simulink model "drone_sine_text"  (R2019a)
settings: Solver=VariableStepAuto  StartTime=0.0  StopTime=inf  RelTol=1e-3
libraries: robotlib x2, aerolibanimutils x1
settings Model: Creator=flying  LastModifiedBy=flying

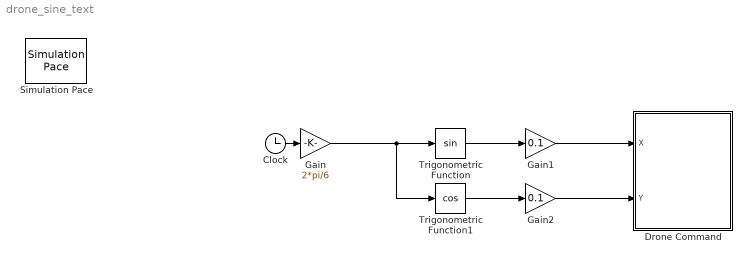
== system drone_sine_text ==
  Clock : Clock
  Drone Command : Subsystem
  Gain : Gain  Gain=2*pi/6
  Gain1 : Gain  Gain=0.1
  Gain2 : Gain  Gain=0.1
  Simulation Pace : aerolibanimutils/Simulation Pace  SimulationPace=1  SleepMode=Auto  OutputPaceError=off  SampleTime=1/30
  Trigonometric Function : Trigonometry
  Trigonometric Function1 : Trigonometry  Operator=cos
  wires:
  Gain/1 -> Trigonometric Function1/1, Trigonometric Function/1
  Clock/1 -> Gain/1
  Trigonometric Function/1 -> Gain1/1
  Trigonometric Function1/1 -> Gain2/1
  Gain1/1 -> Drone Command/1(X)
  Gain2/1 -> Drone Command/2(Y)

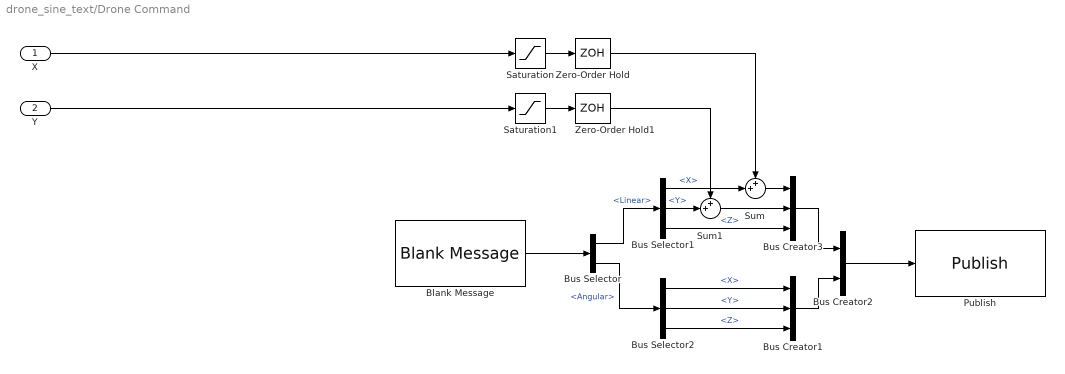
== system drone_sine_text/Drone Command ==
  X : Inport
  Y : Inport  Port=2
  Blank Message : robotlib/Blank Message  messageClass=Message  entityType=geometry_msgs/Twist  messageType=geometry_msgs/Twist  SampleTime=0.0333333333333333333333333
      settings: SourceProductBaseCode=RO
  Bus Creator1 : BusCreator  Inputs=3  OutDataTypeStr=Bus: SL_Bus_drone_sine_text_geometry_msgs_Vector3  NonVirtualBus=on
      settings: InheritFromInputs=off
  Bus Creator2 : BusCreator  Inputs=2  OutDataTypeStr=Bus: SL_Bus_drone_sine_text_geometry_msgs_Twist  NonVirtualBus=on
      settings: InheritFromInputs=off
  Bus Creator3 : BusCreator  Inputs=3  OutDataTypeStr=Bus: SL_Bus_drone_sine_text_geometry_msgs_Vector3  NonVirtualBus=on
      settings: InheritFromInputs=off
  Bus Selector : BusSelector  OutputSignals=Linear,Angular
  Bus Selector1 : BusSelector  OutputSignals=X,Y,Z
  Bus Selector2 : BusSelector  OutputSignals=X,Y,Z
  Publish : robotlib/Publish  topicSource=Select from ROS network  topic=/ext_vel  messageType=geometry_msgs/Twist  messageQueueLength=1
      settings: SourceProductBaseCode=RO
  Saturation : Saturate  UpperLimit=0.1  LowerLimit=-0.1
  Saturation1 : Saturate  UpperLimit=0.1  LowerLimit=-0.1
  Sum : Sum  Inputs=++|
  Sum1 : Sum  Inputs=++|
  Zero-Order Hold : ZeroOrderHold  SampleTime=-1
  Zero-Order Hold1 : ZeroOrderHold  SampleTime=-1
  wires:
  Zero-Order Hold/1 -> Sum/1
  Zero-Order Hold1/1 -> Sum1/1
  Bus Creator1/1 -> Bus Creator2/2
  Sum1/1 -> Bus Creator3/2
  Bus Selector/1 -> Bus Selector1/1  "<Linear>"
  Bus Selector1/2 -> Sum1/2  "<Y>"
  Saturation/1 -> Zero-Order Hold/1
  Bus Selector1/3 -> Bus Creator3/3  "<Z>"
  Saturation1/1 -> Zero-Order Hold1/1
  Bus Creator3/1 -> Bus Creator2/1
  X/1 -> Saturation/1
  Sum/1 -> Bus Creator3/1
  Y/1 -> Saturation1/1
  Bus Selector2/1 -> Bus Creator1/1  "<X>"
  Bus Selector1/1 -> Sum/2  "<X>"
  Bus Creator2/1 -> Publish/1
  Bus Selector2/2 -> Bus Creator1/2  "<Y>"
  Blank Message/1 -> Bus Selector/1
  Bus Selector2/3 -> Bus Creator1/3  "<Z>"
  Bus Selector/2 -> Bus Selector2/1  "<Angular>"
